simulink model "test_plant_A_2015B"  (R2015b)
settings: Solver=VariableStepAuto  StartTime=0.0  StopTime=sim_run  FixedStep=0.001  RelTol=1e-3
undefined symbols (not defined in the file): Standard_Devices, UDP_Protocol, zh_step
libraries: sldrtlib x2, dspnetwork x1
settings Model: Creator=Anony  LastModifiedBy=Anony

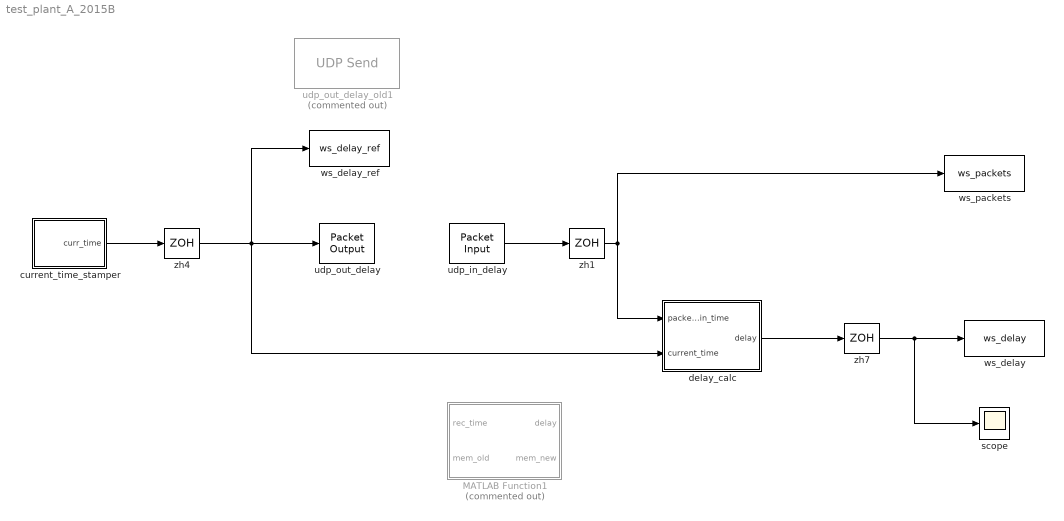
== system test_plant_A_2015B ==
  MATLAB Function1 : MATLAB Function  Commented=on  TreatAsAtomicUnit=on
  current_time_stamper : MATLAB Function  TreatAsAtomicUnit=on
  delay_calc : Subsystem
  scope : Scope
  udp_in_delay : sldrtlib/Packet Input  SampleTime=0.001  MaxMissedTicks=inf  ShowMissedTicks=off  YieldWhenWaiting=off  DrvName=Standard_Devices/UDP_Protocol  DrvAddress=27000  DrvOptions=[2468394756 27000]  PacketSize=8  DataTypes='double'  ShowReady=off  ShowError=off  PacketID=1  ByteOrder=1  ShowTimestamp=off
      settings: AttributesFormatString=Standard Devices\nUDP Protocol [6978h]
  udp_out_delay : sldrtlib/Packet Output  SampleTime=0.01  MaxMissedTicks=inf  ShowMissedTicks=off  YieldWhenWaiting=off  DrvName=Standard_Devices/UDP_Protocol  DrvAddress=28000  DrvOptions=[2468394756 28000]  PacketSize=8  DataTypes='double'  ShowReady=off  ShowError=off  PacketID=1  ByteOrder=1  InitialValue=[]  FinalValue=[]
      settings: AttributesFormatString=Standard Devices\nUDP Protocol [6D6Ah]
  udp_out_delay_old1 : dspnetwork/UDP Send  Commented=on  remoteURL='147.32.183.50'  remotePort=27010  localURL='0.0.0.0'  localPortSource=Automatically determine  localPort=27000  sampletime=-1  separateLengthPort=0
  ws_delay : ToWorkspace  VariableName=ws_delay  SaveFormat=Timeseries  SampleTime=-1
  ws_delay_ref : ToWorkspace  VariableName=ws_delay_ref  SaveFormat=Timeseries  SampleTime=-1
  ws_packets : ToWorkspace  VariableName=ws_packets  SaveFormat=Timeseries  SampleTime=-1
  zh1 : ZeroOrderHold  SampleTime=zh_step
  zh4 : ZeroOrderHold  SampleTime=zh_step
  zh7 : ZeroOrderHold  SampleTime=zh_step
  wires:
  zh4/1 -> delay_calc/2(current_time), ws_delay_ref/1, udp_out_delay/1
  current_time_stamper/1(curr_time) -> zh4/1
  udp_in_delay/1 -> zh1/1
  zh1/1 -> delay_calc/1(packet_in_time), ws_packets/1
  zh7/1 -> scope/1, ws_delay/1
  delay_calc/1(delay) -> zh7/1

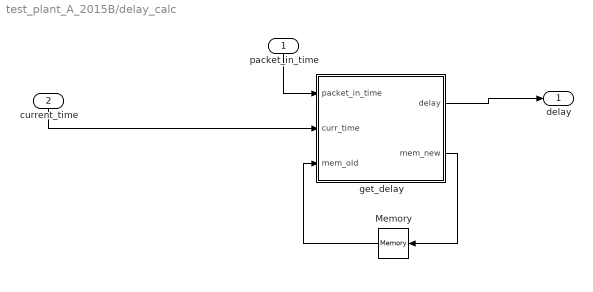
== system test_plant_A_2015B/delay_calc ==
  packet_in_time : Inport
  current_time : Inport  Port=2
  Memory : Memory
  get_delay : MATLAB Function  TreatAsAtomicUnit=on
  delay : Outport
  wires:
  get_delay/2(mem_new) -> Memory/1
  get_delay/1(delay) -> delay/1
  Memory/1 -> get_delay/3(mem_old)
  current_time/1 -> get_delay/2(curr_time)
  packet_in_time/1 -> get_delay/1(packet_in_time)

== matlab function test_plant_A_2015B/current_time_stamper ==
  data: curr_time output
function curr_time = fcn()
%#codegen

coder.extrinsic('get_current_time'); 

     
% pause(0.01);
curr_time = 0;
curr_time = get_current_time();

== matlab function test_plant_A_2015B/MATLAB Function1 ==
  data: delay output; rec_time input; mem_old input; mem_new output
function [delay,mem_new] = fcn(rec_time, mem_old)
%#codegen

coder.extrinsic('get_delay');

delay = 0;
mem_new = 0;

if(rec_time > 0)
    mem_new = rec_time;
    if(mem_old ~= rec_time)
        %         0
        %         rec_time
        delay = get_delay(rec_time); % disp in milisecs
        %         0
    else
        delay = -2; % losst packet
    end
else
    delay = -1;
    
end

== matlab function test_plant_A_2015B/delay_calc/get_delay ==
  data: delay output; packet_in_time input; curr_time input; mem_old input; mem_new output
function [delay,mem_new] = fcn(packet_in_time,...
                               curr_time,...
                               mem_old)
%#codegen

mem_new = 0;

if(packet_in_time > 0)
    mem_new = packet_in_time;
    if(mem_old ~= packet_in_time)
        delay = curr_time - packet_in_time;
    else
        delay = 0; % losst packet 
    end
else
    delay = -5; % no input received
    
end
